simulink model "Punto_3"  (R2025b)
settings: Solver=VariableStepAuto  StartTime=0.0  StopTime=1000  RelTol=1e-3
values from neighbouring files (symbols this model uses):
  ki1 = 0.0055    [Punto_3_Cod.m]
  ki2 = 0.000065    (= 6.5e-05)    [Punto_3_Cod.m]
  ki3 = 0.000000385    (= 3.85e-07)    [Punto_3_Cod.m]
  kp = -8405.61    [Punto_1_Cod.m]    (also in Punto_3_Cod.m = 0.114)
  q0 = (kd/T) + kp + (ki*T)    (= -8302.70879163)    [Punto_1_Cod.m]    (also in Punto_3_Cod.m = 0.62989408)
  q1 = - (2*kd/T) - kp    (= 8356.70054326)    [Punto_1_Cod.m]    (also in Punto_3_Cod.m = -1.08976)
  q2 = kd/T    (= 24.4547283702)    [Punto_1_Cod.m]    (also in Punto_3_Cod.m = 0.628)
  q3 = kp    (= 0.114)    [Punto_3_Cod.m]
  T = 1.988    [Punto_1_Cod.m]    (also in Punto_3_Cod.m = 52)
libraries: simulink x2
settings Model: Creator=Andres Felipe  LastModifiedBy=Andres Felipe

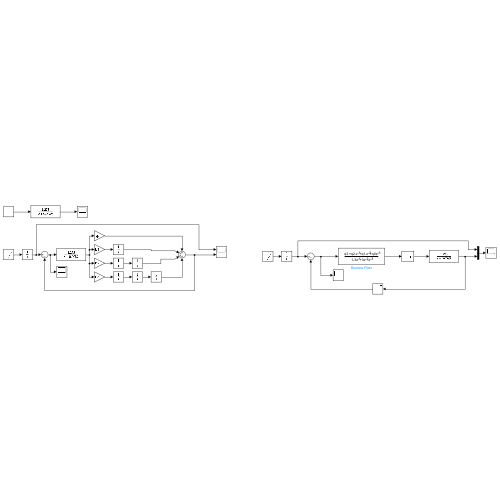
[thumbnail: Simulink's stored preview of the top-level diagram]
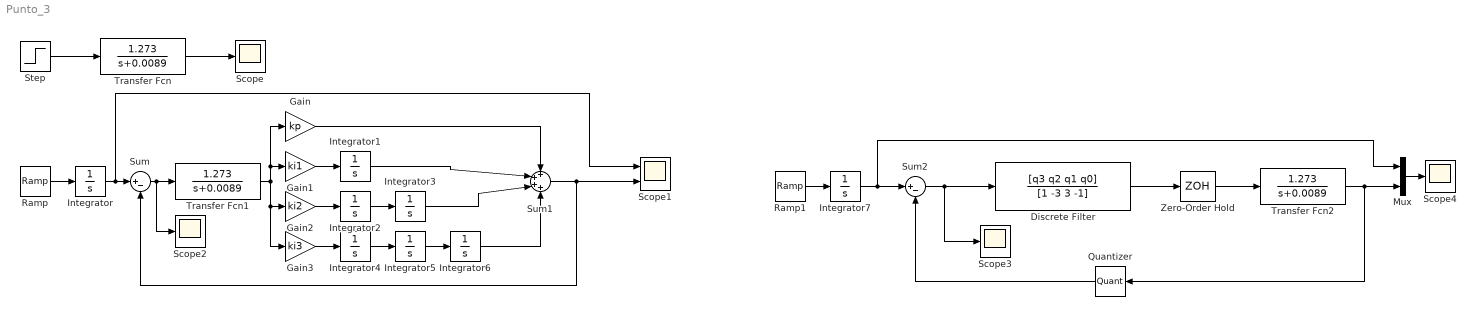
== system Punto_3 ==
  Discrete Filter : DiscreteFilter  Numerator=[q3 q2 q1 q0]  Denominator=[1 -3 3 -1]
  Gain : Gain  Gain=kp
  Gain1 : Gain  Gain=ki1
  Gain2 : Gain  Gain=ki2
  Gain3 : Gain  Gain=ki3
  Integrator{,1..7} (8 alike) : Integrator
  Mux : Mux  Inputs=2
  Quantizer : Quantizer  QuantizationInterval=3.3/4095
  Ramp : simulink/Sources/Ramp  slope=1  start=0  InitialOutput=0
  Ramp1 : simulink/Sources/Ramp  slope=1  start=0  InitialOutput=0
  Scope{,2..4} (4 alike) : Scope
      Scope settings: ActiveDisplayYMinimum=-1  ActiveDisplayYMaximum=1
      Scope2 settings: ActiveDisplayYMinimum=-1  ActiveDisplayYMaximum=1  DataLoggingVariableName=ScopeData2
      Scope3 settings: ActiveDisplayYMinimum=-1  ActiveDisplayYMaximum=1  DataLoggingVariableName=ScopeData3
      Scope4 settings: ActiveDisplayYMinimum=-1  ActiveDisplayYMaximum=1  DataLoggingVariableName=ScopeData4
  Scope1 : Scope  NumInputPorts=2
      settings: ActiveDisplayYMinimum=-1  ActiveDisplayYMaximum=1
  Step : Step  Time=0  SampleTime=0
  Sum : Sum  Inputs=|+-
  Sum1 : Sum  Inputs=++++
  Sum2 : Sum  Inputs=|+-
  Transfer Fcn : TransferFcn  Numerator=[1.273]  Denominator=[1 0.0089]
  Transfer Fcn1 : TransferFcn  Numerator=[1.273]  Denominator=[1 0.0089]
  Transfer Fcn2 : TransferFcn  Numerator=[1.273]  Denominator=[1 0.0089]
  Zero-Order Hold : ZeroOrderHold  SampleTime=T
  wires:
  Transfer Fcn/1 -> Scope/1
  Step/1 -> Transfer Fcn/1
  Ramp/1 -> Integrator/1
  Integrator/1 -> Scope1/1, Sum/1
  Sum/1 -> Scope2/1, Transfer Fcn1/1
  Transfer Fcn1/1 -> Gain3/1, Gain2/1, Gain/1, Gain1/1
  Gain1/1 -> Integrator1/1
  Gain2/1 -> Integrator2/1
  Integrator2/1 -> Integrator3/1
  Integrator4/1 -> Integrator5/1
  Integrator5/1 -> Integrator6/1
  Gain3/1 -> Integrator4/1
  Gain/1 -> Sum1/1
  Integrator1/1 -> Sum1/2
  Integrator3/1 -> Sum1/3
  Integrator6/1 -> Sum1/4
  Sum1/1 -> Sum/2, Scope1/2
  Sum2/1 -> Scope3/1, Discrete Filter/1
  Zero-Order Hold/1 -> Transfer Fcn2/1
  Quantizer/1 -> Sum2/2
  Discrete Filter/1 -> Zero-Order Hold/1
  Integrator7/1 -> Sum2/1, Mux/1
  Transfer Fcn2/1 -> Mux/2, Quantizer/1
  Ramp1/1 -> Integrator7/1
  Mux/1 -> Scope4/1
